simulink model "ReactionJetControl"  (R2021a)
settings: configuration reference "CSRef" (kept outside this file)
undefined symbols (not defined in the file): delt
settings Model: Creator=pkhetarp  LastModifiedBy=pkhetarp
settings ConfigSetRef: SourceName=CSRef  SourceLocation=Base Workspace

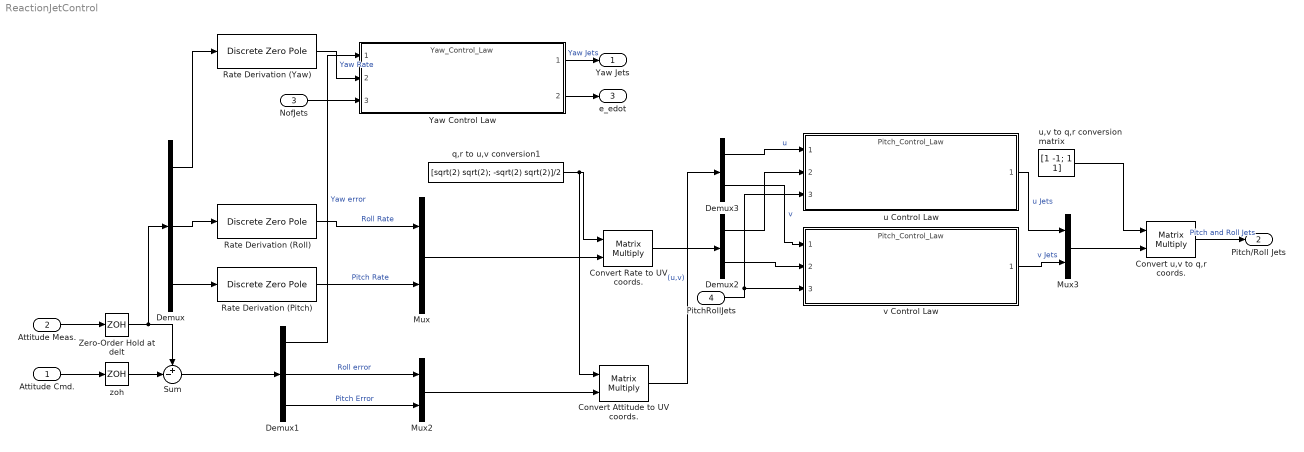
== system ReactionJetControl ==
  Attitude Cmd. : Inport  Unit=rad  PortDimensions=[1 3]
  Attitude Meas. : Inport  Port=2  Unit=rad
  NofJets : Inport  Port=3
  PitchRollJets : Inport  Port=4
  Convert Attitude to UV coords. : Product  Multiplication=Matrix(*)  InputSameDT=on  RndMeth=Zero  SaturateOnIntegerOverflow=on  OutDataTypeStr=Inherit: Same as first input
  Convert Rate to UV coords. : Product  Multiplication=Matrix(*)  InputSameDT=on  RndMeth=Zero  SaturateOnIntegerOverflow=on  OutDataTypeStr=Inherit: Same as first input
  Convert u,v to q,r coords. : Product  Multiplication=Matrix(*)  InputSameDT=on  RndMeth=Zero  SaturateOnIntegerOverflow=on  OutDataTypeStr=Inherit: Same as first input
  Demux : Demux  Outputs=3
      settings: DisplayOption=none
  Demux1 : Demux  Outputs=3
      settings: DisplayOption=none
  Demux2 : Demux  Outputs=2
      settings: DisplayOption=none
  Demux3 : Demux  Outputs=2
      settings: DisplayOption=none
  Mux : Mux  Inputs=2
  Mux2 : Mux  Inputs=2
  Mux3 : Mux  Inputs=2
  Rate Derivation (Pitch) : DiscreteZeroPole  Poles=[0]  Gain=1/delt  SampleTime=-1
  Rate Derivation (Roll) : DiscreteZeroPole  Poles=[0]  Gain=1/delt  SampleTime=-1
  Rate Derivation (Yaw) : DiscreteZeroPole  Poles=[0]  Gain=1/delt  SampleTime=-1
  Sum : Sum  Inputs=+-|  InputSameDT=on  SaturateOnIntegerOverflow=on  OutDataTypeStr=Inherit: Same as first input
  Yaw Control Law : ModelReference  ModelNameDialog=Yaw_Control_Law  UsingDefaultArgumentValue=0,0  ModelReferenceVersion=1.13  alph=alph1  alphs=alphs1
  Zero-Order Hold at delt : ZeroOrderHold  SampleTime=delt
  q,r to u,v conversion1 : Constant  Value=[sqrt(2) sqrt(2); -sqrt(2) sqrt(2)]/2  VectorParams1D=off
  u Control Law : ModelReference  ModelNameDialog=Pitch_Control_Law  UsingDefaultArgumentValue=0,0  ModelReferenceVersion=1.10  alph=alphu  alphs=alphsu
  u,v to q,r conversion matrix : Constant  Value=[1 -1; 1 1]  VectorParams1D=off
  v Control Law : ModelReference  ModelNameDialog=Pitch_Control_Law  UsingDefaultArgumentValue=0,0  ModelReferenceVersion=1.10  alph=alphv  alphs=alphsv
  zoh : ZeroOrderHold  SampleTime=delt
  Yaw Jets : Outport  Unit=lbf  OutputWhenDisabled=reset  InitialOutput=0  VectorParamsAs1DForOutWhenUnconnected=off
  Pitch/Roll Jets : Outport  Port=2  Unit=lbf  OutputWhenDisabled=reset  InitialOutput=0  VectorParamsAs1DForOutWhenUnconnected=off
  e_edot : Outport  Port=3
  wires:
  Demux/1 -> Rate Derivation (Yaw)/1
  Rate Derivation (Roll)/1 -> Mux/1  "Roll Rate"
  Demux/3 -> Rate Derivation (Pitch)/1
  Rate Derivation (Pitch)/1 -> Mux/2  "Pitch Rate"
  Demux2/2 -> v Control Law/2
  Demux/2 -> Rate Derivation (Roll)/1
  Mux/1 -> Convert Rate to UV coords./2
  Demux1/2 -> Mux2/1  "Roll error"
  u Control Law/1 -> Mux3/1  "u Jets"
  PitchRollJets/1 -> v Control Law/3, u Control Law/3
  Rate Derivation (Yaw)/1 -> Yaw Control Law/2  "Yaw Rate"
  Demux1/1 -> Yaw Control Law/1  "Yaw error"
  q,r to u,v conversion1/1 -> Convert Rate to UV coords./1, Convert Attitude to UV coords./1
  Demux3/2 -> v Control Law/1  "v"
  Attitude Meas./1 -> Zero-Order Hold at delt/1
  Convert Attitude to UV coords./1 -> Demux3/1  "(u,v)"
  zoh/1 -> Sum/2
  Convert u,v to q,r coords./1 -> Pitch/Roll Jets/1  "Pitch and Roll Jets"
  v Control Law/1 -> Mux3/2  "v Jets"
  Attitude Cmd./1 -> zoh/1
  Sum/1 -> Demux1/1
  Demux1/3 -> Mux2/2  "Pitch Error"
  Convert Rate to UV coords./1 -> Demux2/1
  NofJets/1 -> Yaw Control Law/3
  Zero-Order Hold at delt/1 -> Demux/1, Sum/1
  u,v to q,r conversion matrix/1 -> Convert u,v to q,r coords./1
  Yaw Control Law/2 -> e_edot/1
  Demux2/1 -> u Control Law/2
  Demux3/1 -> u Control Law/1  "u"
  Mux3/1 -> Convert u,v to q,r coords./2
  Yaw Control Law/1 -> Yaw Jets/1  "Yaw Jets"
  Mux2/1 -> Convert Attitude to UV coords./2
